simulink model "nonlin_sim"  (R2023a)
settings: Solver=VariableStepAuto  StartTime=0.0  StopTime=10  RelTol=1e-3
values from neighbouring files (symbols this model uses):
  A_lin = double(subs(jacobian(f, [x1, x2, x3, x4]), all_variables, all_values))    [nonlin_lab.m]    (also in nonlin_lab_task2.m; nonlin_lab_task4.m; nonlin_lab_task6.m)
  B_lin = double(subs(jacobian(f, nu), all_variables, all_values))    [nonlin_lab.m]    (also in nonlin_lab_task2.m; nonlin_lab_task4.m; nonlin_lab_task6.m)
  C = [1 1 1 1]    [nonlin_lab.m]    (also in nonlin_lab_task2.m = [1 0 1 0]; nonlin_lab_task4.m = [1 0 0 0]; nonlin_lab_task6.m = [1 0 0 0])
  K = K_aug(1:4)    [nonlin_lab.m]    (also in nonlin_lab_task2.m)
  K_2 = K_aug(1:4)    [nonlin_lab_task4.m]    (also in nonlin_lab_task6.m)
  K_ff = pinv(B_lin)    [nonlin_lab.m]    (also in nonlin_lab_task2.m)
  K_i = 10*abs(K_aug(5))    [nonlin_lab.m]    (also in nonlin_lab_task2.m = 1*abs(K_aug(5)); nonlin_lab_task4.m = 1*abs(K_aug(5)); nonlin_lab_task6.m = 1*abs(K_aug(5)))
  K_poles = place(A_lin, B_lin, poles)    [nonlin_lab_task4.m]    (also in nonlin_lab_task6.m)
  La_La_La_La_c_at_x0_numeric = double(subs(La_La_La_La_c_at_x0, param_values, param_numeric))    [nonlin_lab_task4.m]    (also in nonlin_lab_task6.m)
  Lb_La_La_La_c_at_x0_numeric = double(subs(Lb_La_La_La_c_at_x0, param_values, param_numeric))    [nonlin_lab_task4.m]    (also in nonlin_lab_task6.m)
  x_init = [0 0 0 0]'    [nonlin_lab.m]    (also in nonlin_lab_task2.m = [0 0 theta_m_eq 0]'; nonlin_lab_task4.m = [0 0 theta_m_eq 0]'; nonlin_lab_task6.m = [0 0 theta_m_eq 0]')
  x_ref = [pi/4; 0 ; 0; 0]    [nonlin_lab.m]    (also in nonlin_lab_task2.m = [theta_l_eq 0 theta_m_eq 0]'; nonlin_lab_task4.m = [theta_l_eq 0 theta_m_eq 0]'; nonlin_lab_task6.m = [theta_l_eq 0 theta_m_eq 0]')
undefined symbols (not defined in the file or in its folder): K_lin_feedback
settings Model: Creator=M4RTI  LastModifiedBy=M4RTI

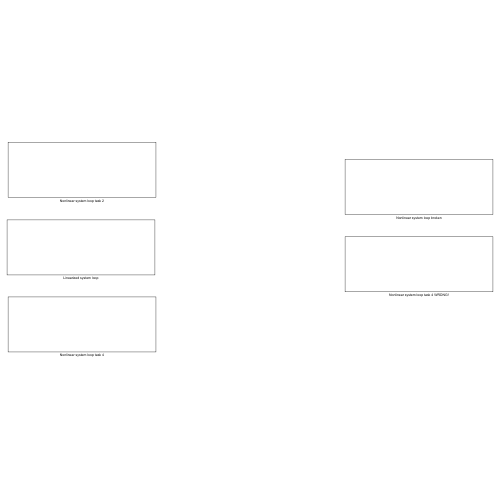
[thumbnail: Simulink's stored preview of the top-level diagram]
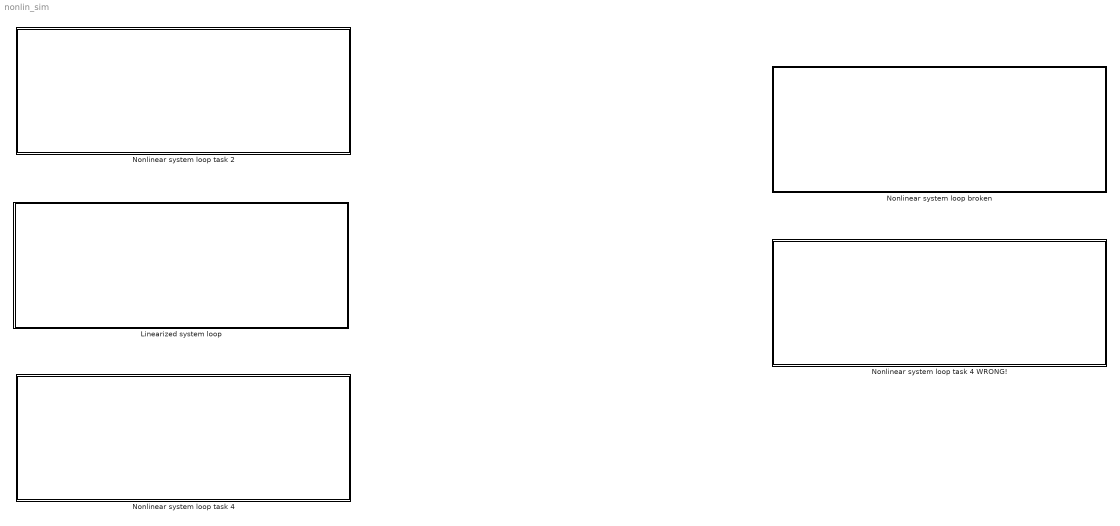
== system nonlin_sim ==
  Linearized system loop : Subsystem
  Nonlinear system loop broken : Subsystem
  Nonlinear system loop task 2 : Subsystem
  Nonlinear system loop task 4 : Subsystem
  Nonlinear system loop task 4 WRONG! : Subsystem

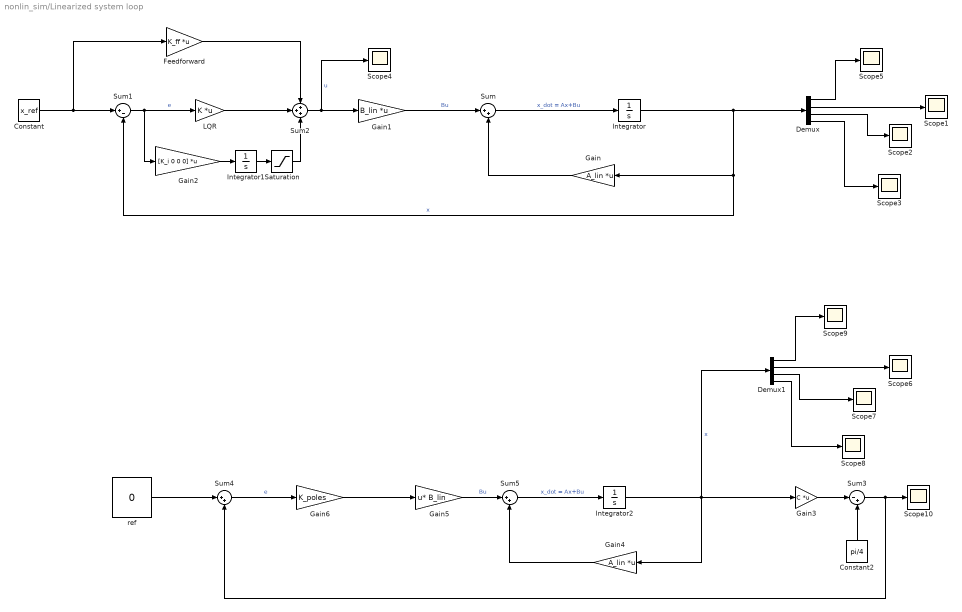
== system nonlin_sim/Linearized system loop ==
  Constant : Constant  Value=x_ref  VectorParams1D=off
  Constant2 : Constant  Value=pi/4
  Demux : Demux
  Demux1 : Demux
  Feedforward : Gain  Gain=K_ff  Multiplication=Matrix(K*u)
  Gain : Gain  Gain=A_lin  Multiplication=Matrix(K*u)
  Gain1 : Gain  Gain=B_lin  Multiplication=Matrix(K*u)
  Gain2 : Gain  Gain=[K_i 0 0 0]  Multiplication=Matrix(K*u)
  Gain3 : Gain  Gain=C  Multiplication=Matrix(K*u)
  Gain4 : Gain  Gain=A_lin  Multiplication=Matrix(K*u)
  Gain5 : Gain  Gain=B_lin  Multiplication=Matrix(u*K)
  Gain6 : Gain  Gain=K_poles
  Integrator : Integrator  InitialCondition=x_init
  Integrator1 : Integrator
  Integrator2 : Integrator  InitialCondition=x_init
  LQR : Gain  Gain=K  Multiplication=Matrix(K*u)
  Saturation : Saturate  UpperLimit=5  LowerLimit=-5
  Scope{1..10} (10 alike) : Scope
  Sum : Sum  Inputs=|++
  Sum1 : Sum  Inputs=|+-
  Sum2 : Sum  Inputs=+++
  Sum3 : Sum  Inputs=|-+
  Sum4 : Sum  Inputs=|++
  Sum5 : Sum  Inputs=|++
  ref : Constant  Value=0  VectorParams1D=off
  wires:
  Demux/2 -> Scope1/1
  LQR/1 -> Sum2/2
  Sum/1 -> Integrator/1  "x_dot = Ax+Bu"
  Integrator/1 -> Demux/1, Sum1/2, Gain/1  "x"
  Gain/1 -> Sum/2
  Demux/1 -> Scope5/1
  Gain1/1 -> Sum/1  "Bu"
  Sum1/1 -> LQR/1, Gain2/1  "e"
  Demux/3 -> Scope2/1
  Demux/4 -> Scope3/1
  Constant/1 -> Feedforward/1, Sum1/1
  Sum2/1 -> Scope4/1, Gain1/1  "u"
  Feedforward/1 -> Sum2/1
  Gain2/1 -> Integrator1/1
  Integrator1/1 -> Saturation/1
  Saturation/1 -> Sum2/3
  Integrator2/1 -> Gain4/1, Gain3/1, Demux1/1  "x"
  Sum3/1 -> Sum4/2, Scope10/1
  Constant2/1 -> Sum3/2
  Demux1/4 -> Scope8/1
  Gain3/1 -> Sum3/1
  Demux1/2 -> Scope6/1
  Demux1/3 -> Scope7/1
  Demux1/1 -> Scope9/1
  Gain4/1 -> Sum5/2
  Gain5/1 -> Sum5/1  "Bu"
  Sum5/1 -> Integrator2/1  "x_dot = Ax+Bu"
  ref/1 -> Sum4/1
  Sum4/1 -> Gain6/1  "e"
  Gain6/1 -> Gain5/1

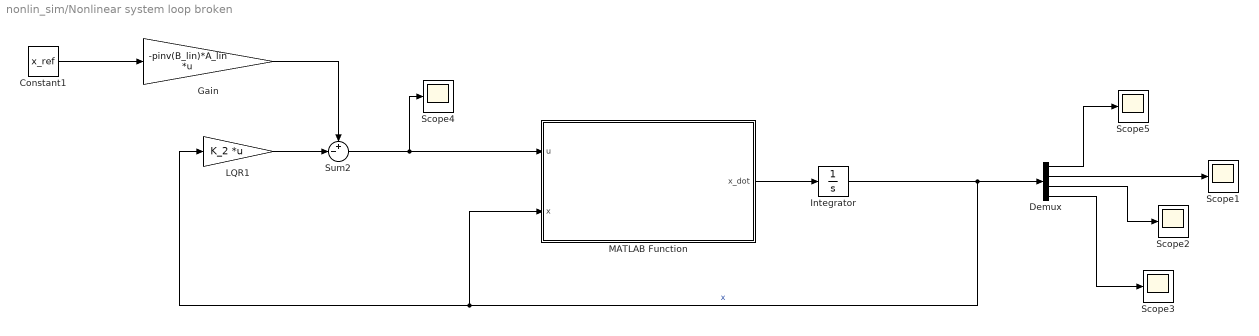
== system nonlin_sim/Nonlinear system loop broken ==
  Constant1 : Constant  Value=x_ref
  Demux : Demux
  Gain : Gain  Gain=-pinv(B_lin)*A_lin  Multiplication=Matrix(K*u)
  Integrator : Integrator  InitialCondition=x_init
  LQR1 : Gain  Gain=K_2  Multiplication=Matrix(K*u)
  MATLAB Function : MATLAB Function  TreatAsAtomicUnit=on
  Scope{1..5} (5 alike) : Scope
  Sum2 : Sum  Inputs=+-|
  wires:
  Demux/1 -> Scope5/1
  Demux/4 -> Scope3/1
  Demux/2 -> Scope1/1
  Demux/3 -> Scope2/1
  MATLAB Function/1(x_dot) -> Integrator/1
  Integrator/1 -> Demux/1, LQR1/1, MATLAB Function/2(x)  "x"
  Constant1/1 -> Gain/1
  Sum2/1 -> Scope4/1, MATLAB Function/1(u)
  LQR1/1 -> Sum2/2
  Gain/1 -> Sum2/1

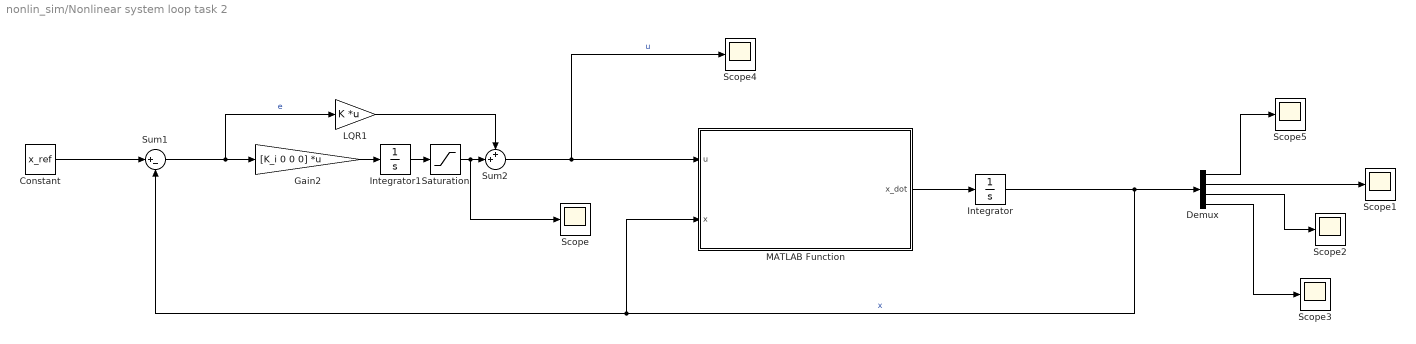
== system nonlin_sim/Nonlinear system loop task 2 ==
  Constant : Constant  Value=x_ref  VectorParams1D=off
  Demux : Demux
  Gain2 : Gain  Gain=[K_i 0 0 0]  Multiplication=Matrix(K*u)
  Integrator : Integrator  InitialCondition=x_init
  Integrator1 : Integrator
  LQR1 : Gain  Gain=K  Multiplication=Matrix(K*u)
  MATLAB Function : MATLAB Function  TreatAsAtomicUnit=on
  Saturation : Saturate  UpperLimit=100  LowerLimit=-100
  Scope{,1..5} (6 alike) : Scope
  Sum1 : Sum  Inputs=|+-
  Sum2 : Sum  Inputs=++|
  wires:
  Constant/1 -> Sum1/1
  Demux/1 -> Scope5/1
  Demux/4 -> Scope3/1
  Integrator/1 -> Demux/1, MATLAB Function/2(x), Sum1/2  "x"
  Demux/2 -> Scope1/1
  Demux/3 -> Scope2/1
  MATLAB Function/1(x_dot) -> Integrator/1
  Integrator1/1 -> Saturation/1
  Saturation/1 -> Scope/1, Sum2/2
  Gain2/1 -> Integrator1/1
  Sum2/1 -> MATLAB Function/1(u), Scope4/1  "u"
  LQR1/1 -> Sum2/1
  Sum1/1 -> Gain2/1, LQR1/1  "e"

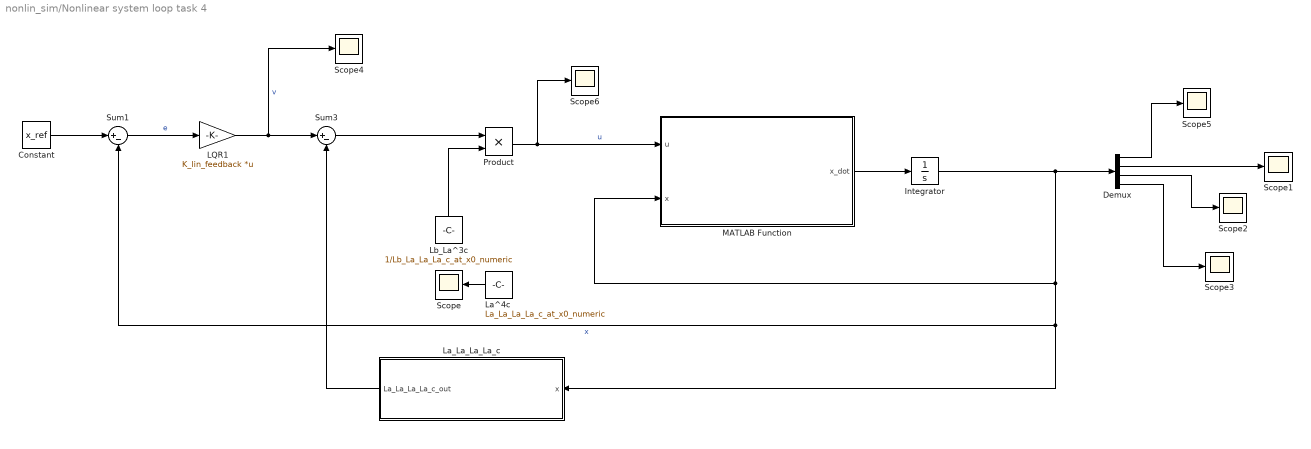
== system nonlin_sim/Nonlinear system loop task 4 ==
  Constant : Constant  Value=x_ref  VectorParams1D=off
  Demux : Demux
  Integrator : Integrator  InitialCondition=x_init
  LQR1 : Gain  Gain=K_lin_feedback  Multiplication=Matrix(K*u)
  La^4c : Constant  Value=La_La_La_La_c_at_x0_numeric
  La_La_La_La_c : MATLAB Function  TreatAsAtomicUnit=on
  Lb_La^3c : Constant  Value=1/Lb_La_La_La_c_at_x0_numeric
  MATLAB Function : MATLAB Function  TreatAsAtomicUnit=on
  Product : Product
  Scope{,1..6} (7 alike) : Scope
  Sum1 : Sum  Inputs=|+-
  Sum3 : Sum  Inputs=|+-
  wires:
  Constant/1 -> Sum1/1
  Demux/1 -> Scope5/1
  Demux/4 -> Scope3/1
  Integrator/1 -> Demux/1, MATLAB Function/2(x), Sum1/2, La_La_La_La_c/1(x)  "x"
  Demux/2 -> Scope1/1
  Demux/3 -> Scope2/1
  MATLAB Function/1(x_dot) -> Integrator/1
  Sum1/1 -> LQR1/1  "e"
  Product/1 -> Scope6/1, MATLAB Function/1(u)  "u"
  LQR1/1 -> Scope4/1, Sum3/1  "v"
  Sum3/1 -> Product/1
  Lb_La^3c/1 -> Product/2
  La^4c/1 -> Scope/1
  La_La_La_La_c/1(La_La_La_La_c_out) -> Sum3/2

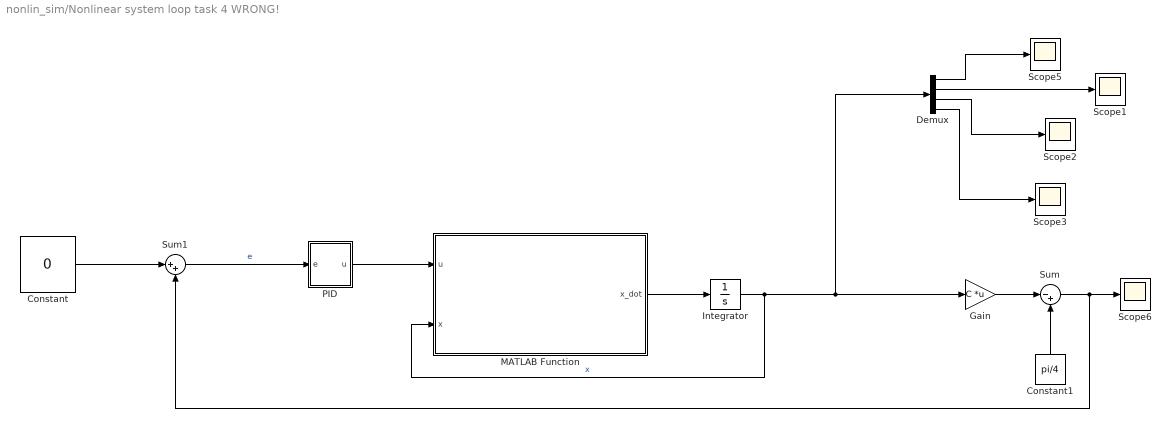
== system nonlin_sim/Nonlinear system loop task 4 WRONG! ==
  Constant : Constant  Value=0  VectorParams1D=off
  Constant1 : Constant  Value=pi/4
  Demux : Demux
  Gain : Gain  Gain=C  Multiplication=Matrix(K*u)
  Integrator : Integrator  InitialCondition=x_init
  MATLAB Function : MATLAB Function  TreatAsAtomicUnit=on
  PID : Subsystem
  Scope{1..3,5..6} (5 alike) : Scope
  Sum : Sum  Inputs=|-+
  Sum1 : Sum  Inputs=|++
  wires:
  Constant/1 -> Sum1/1
  Demux/1 -> Scope5/1
  Demux/4 -> Scope3/1
  Integrator/1 -> Gain/1, Demux/1, MATLAB Function/2(x)  "x"
  Demux/2 -> Scope1/1
  Demux/3 -> Scope2/1
  MATLAB Function/1(x_dot) -> Integrator/1
  Constant1/1 -> Sum/2
  Gain/1 -> Sum/1
  Sum/1 -> Sum1/2, Scope6/1
  Sum1/1 -> PID/1(e)  "e"
  PID/1(u) -> MATLAB Function/1(u)

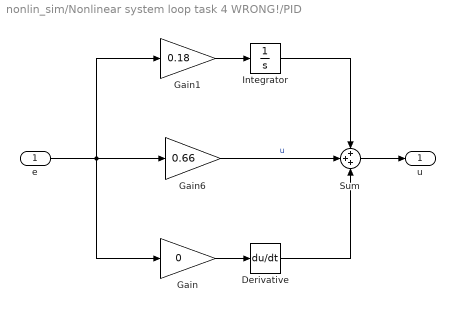
== system nonlin_sim/Nonlinear system loop task 4 WRONG!/PID ==
  e : Inport
  Derivative : Derivative
  Gain : Gain  Gain=0
  Gain1 : Gain  Gain=0.18
  Gain6 : Gain  Gain=0.66
  Integrator : Integrator
  Sum : Sum  Inputs=+++
  u : Outport
  wires:
  e/1 -> Gain1/1, Gain/1, Gain6/1
  Gain/1 -> Derivative/1
  Sum/1 -> u/1
  Integrator/1 -> Sum/1
  Derivative/1 -> Sum/3
  Gain6/1 -> Sum/2  "u"
  Gain1/1 -> Integrator/1

== matlab function nonlin_sim/Nonlinear system loop broken/MATLAB Function ==
  data: u input; x input; x_dot output
function x_dot = nonlin_system(u, x)
    m = 0.3;   % Mass of the load (kg)
    l = 0.3;   % Length to the center of mass of the load (m)
    g = 9.8;   % Acceleration due to gravity (m/s^2)
    J_l = 4e-4; % Moment of inertia of the load (Nms^2/rad)
    J_m = 4e-4; % Moment of inertia of the motor (Nms^2/rad)
    B_l = 0.0;  % Damping coefficient of the load (Nms/rad)
    B_m = 0.015; % Damping coefficient of the motor (Nms/rad)
    k = 0.8;    % Spring constant (Nm/rad)

    % Nonlinear dynamics
    theta_l = x(1);
    theta_l_dot = x(2);
    theta_m = x(3);
    theta_m_dot = x(4);

    x1_dot = theta_l_dot;
    x2_dot = -1/J_l * (B_l * theta_l_dot + k * (theta_l - theta_m) + m * g * l * cos(theta_l));
    x3_dot = theta_m_dot;
    x4_dot = 1/J_m * (u + k * (theta_l - theta_m) - B_m * theta_m_dot);

    % Output: the derivatives of the state variables
    x_dot = [x1_dot; x2_dot; x3_dot; x4_dot];
end

== matlab function nonlin_sim/Nonlinear system loop task 2/MATLAB Function ==
  data: u input; x input; x_dot output
function x_dot = nonlin_system(u, x)
    m = 0.3;   % Mass of the load (kg)
    l = 0.3;   % Length to the center of mass of the load (m)
    g = 9.8;   % Acceleration due to gravity (m/s^2)
    J_l = 4e-4; % Moment of inertia of the load (Nms^2/rad)
    J_m = 4e-4; % Moment of inertia of the motor (Nms^2/rad)
    B_l = 0.0;  % Damping coefficient of the load (Nms/rad)
    B_m = 0.015; % Damping coefficient of the motor (Nms/rad)
    k = 0.8;    % Spring constant (Nm/rad)

    % Nonlinear dynamics
    theta_l = x(1);
    theta_l_dot = x(2);
    theta_m = x(3);
    theta_m_dot = x(4);

    x1_dot = theta_l_dot;
    x2_dot = -1/J_l * (B_l * theta_l_dot + k * (theta_l - theta_m) + m * g * l * cos(theta_l));
    x3_dot = theta_m_dot;
    x4_dot = 1/J_m * (u + k * (theta_l - theta_m) - B_m * theta_m_dot);

    % Output: the derivatives of the state variables
    x_dot = [x1_dot; x2_dot; x3_dot; x4_dot];
end

== matlab function nonlin_sim/Nonlinear system loop task 4 WRONG!/MATLAB Function ==
  data: u input; x input; x_dot output
function x_dot = nonlin_system(u, x)
    m = 0.3;   % Mass of the load (kg)
    l = 0.3;   % Length to the center of mass of the load (m)
    g = 9.8;   % Acceleration due to gravity (m/s^2)
    J_l = 4e-4; % Moment of inertia of the load (Nms^2/rad)
    J_m = 4e-4; % Moment of inertia of the motor (Nms^2/rad)
    B_l = 0.0;  % Damping coefficient of the load (Nms/rad)
    B_m = 0.015; % Damping coefficient of the motor (Nms/rad)
    k = 0.8;    % Spring constant (Nm/rad)

    % Nonlinear dynamics
    theta_l = x(1);
    theta_l_dot = x(2);
    theta_m = x(3);
    theta_m_dot = x(4);

    x1_dot = theta_l_dot;
    x2_dot = -1/J_l * (B_l * theta_l_dot + k * (theta_l - theta_m) + m * g * l * cos(theta_l));
    x3_dot = theta_m_dot;
    x4_dot = 1/J_m * (u + k * (theta_l - theta_m) - B_m * theta_m_dot);

    % Output: the derivatives of the state variables
    x_dot = [x1_dot; x2_dot; x3_dot; x4_dot];
end

== matlab function nonlin_sim/Nonlinear system loop task 4/MATLAB Function ==
  data: u input; x input; x_dot output
function x_dot = nonlin_system(u, x)
    m = 0.3;   % Mass of the load (kg)
    l = 0.3;   % Length to the center of mass of the load (m)
    g = 9.8;   % Acceleration due to gravity (m/s^2)
    J_l = 4e-4; % Moment of inertia of the load (Nms^2/rad)
    J_m = 4e-4; % Moment of inertia of the motor (Nms^2/rad)
    B_l = 0.0;  % Damping coefficient of the load (Nms/rad)
    B_m = 0.015; % Damping coefficient of the motor (Nms/rad)
    k = 0.8;    % Spring constant (Nm/rad)

    % Nonlinear dynamics
    theta_l = x(1);
    theta_l_dot = x(2);
    theta_m = x(3);
    theta_m_dot = x(4);

    x1_dot = theta_l_dot;
    x2_dot = -1/J_l * (B_l * theta_l_dot + k * (theta_l - theta_m) + m * g * l * cos(theta_l));
    x3_dot = theta_m_dot;
    x4_dot = 1/J_m * (u + k * (theta_l - theta_m) - B_m * theta_m_dot);

    % Output: the derivatives of the state variables
    x_dot = [x1_dot; x2_dot; x3_dot; x4_dot];
end

== matlab function nonlin_sim/Nonlinear system loop task 4/La_La_La_La_c ==
  data: x input; La_La_La_La_c_out output
function La_La_La_La_c_out = computeLaLaLaLaC(x)
    m = 0.3;   % Mass of the load (kg)
    l = 0.3;   % Length to the center of mass of the load (m)
    g = 9.8;   % Acceleration due to gravity (m/s^2)
    J_l = 4e-4; % Moment of inertia of the load (Nms^2/rad)
    J_m = 4e-4; % Moment of inertia of the motor (Nms^2/rad)
    B_l = 0.0;  % Damping coefficient of the load (Nms/rad)
    B_m = 0.015; % Damping coefficient of the motor (Nms/rad)
    k = 0.8;    % Spring constant (Nm/rad)

    % Extract state variables from x
    theta_l = x(1);
    theta_l_dot = x(2);
    theta_m = x(3);
    theta_m_dot = x(4);

    % Compute La_La_La_La_c
    La_La_La_La_c_out = ((k*(theta_l - theta_m))/J_l + (B_l*theta_l_dot)/J_l + (g*l*m*cos(theta_l))/J_l)*(B_l^2/J_l^2 - k/J_l + (g*l*m*sin(theta_l))/J_l) - theta_l_dot*((B_l*(k/J_l - (g*l*m*sin(theta_l))/J_l))/J_l + (g*l*m*theta_l_dot*cos(theta_l))/J_l) - (k*((k*(theta_l - theta_m))/J_m - (B_m*theta_m_dot)/J_m))/J_l + (B_l*k*theta_m_dot)/J_l^2;
end
